simulink model "AED2D"  (R2018b)
settings: Solver=FixedStepAuto  StartTime=0.0  StopTime=Tfim  FixedStep=0.001  MaxStep=0.001  RelTol=1e-3
values from neighbouring files (symbols this model uses):
  D = DadosCGInercia(D)    [PlotGMax.m]    (also in S.mat = ; VooUnico.m; VooUnico6DOF.m)
  dados =     [S.mat]
  g = 9.8    [plot_exocet_6dof.m]
  M_CD = [8.341 8.24 8.141 8.043 7.946 7.851 7.76 7.674 7.595 7.523 7.46 7.4 ... (1365 elements, 21x5x13)]    [S.mat]
  M_CM = [42.757 43.119 43.498 43.905 44.357 44.839 45.319 45.775 46.191 46.536 46.769 46.963 ... (1365 elements, 21x5x13)]    [S.mat]
  M_CMQ = [-1543.746 -1552.906 -1559.915 -1565.64 -1570.662 -1573.443 -1572.931 -1569.859 -1564.198 -1553.449 -1535.22 -1514.504 ... (1365 elements, 21x5x13)]    [S.mat]
  M_CN = [-21.126 -21.088 -21.046 -20.997 -20.94 -20.877 -20.812 -20.749 -20.692 -20.644 -20.613 -20.587 ... (1365 elements, 21x5x13)]    [S.mat]
  R2D = 57.2957795131    [S.mat]    (also in VooUnico.m; VooUnico6DOF.m; plot6DOF.m; plot_exocet_6dof.m)
undefined symbols (not defined in the file or in its folder): AclnMax, AltCruz, anp, dist_manobra, Dlt_max, Dlt_max_roll, F_propB, F_propS, GanhoAtit, M_CMAD, M_CNAD, M_CNQ, manobra, Newton, ng, p0, phi0, psi0, psimaxAD, q0, r0, RampaMax, Raphson, sat_integAP, sigmaYmaxAD, sigmaZmaxAD, T_acel_k_ext, T_acel_k_int, T_at_k_ext, T_at_k_int, theta0, thetamaxAD, TLaser, Tresp, TTrav, vet_altitude, vet_Mach, vet_x_CG, Vxa0, Vya0, Vza0, Xa0, Ya0, Za0
libraries: simulink x11, sharedutil x4, aerolibasang x4, vrlib x3, shared6dof x2, aerolibatmos2 x1, dspmtrx3 x1
(part 1 of 2)
settings Model: Creator=carlberto-old  LastModifiedBy=carlberto-old
settings SFSimCC: SimUseLocalCustomCode=off
settings RTWCC: RTWUseLocalCustomCode=off

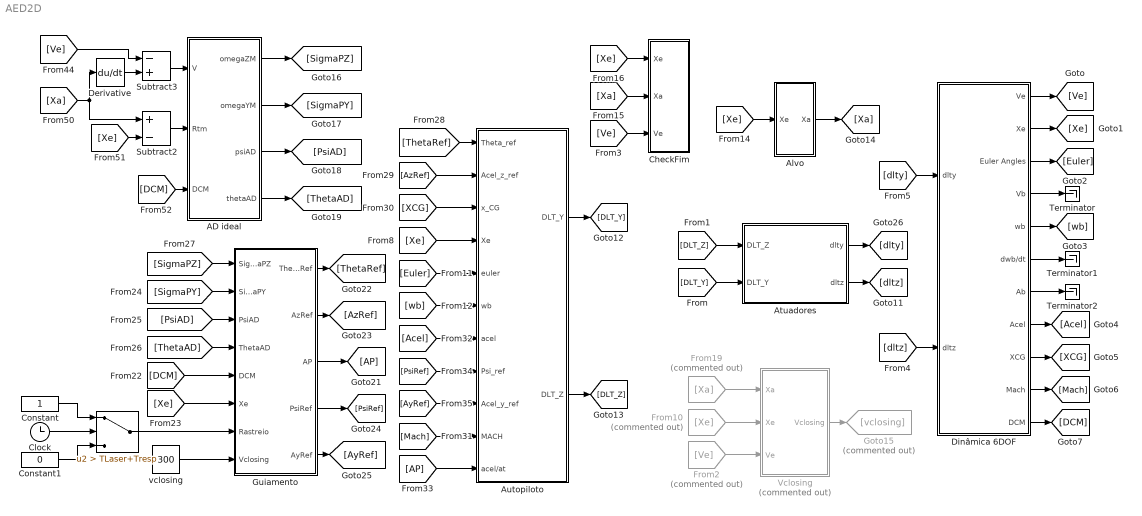
== system AED2D ==
  "  " : Switch  Criteria=u2 > Threshold  Threshold=TLaser+Tresp
  AD ideal : Subsystem
  Alvo : Subsystem
  Atuadores : Subsystem
  Autopiloto : Subsystem
  CheckFim : Subsystem
  Clock : Clock
  Constant : Constant
  Constant1 : Constant  Value=0
  Derivative : Derivative
  Dinâmica 6DOF : Subsystem
  From10 : From  Commented=on  GotoTag=Xe
  From19 : From  Commented=on  GotoTag=Xa
  From2 : From  Commented=on  GotoTag=Ve
  Goto15 : Goto  Commented=on  GotoTag=vclosing
  Guiamento : Subsystem
  Subtract2 : Sum  Inputs=+-
  Subtract3 : Sum  Inputs=-+
  Terminator : Terminator
  Terminator1 : Terminator
  Terminator2 : Terminator
  Vclosing : Subsystem  Commented=on
  vclosing : Constant  Value=300
  wires:
  [dltz] -> Dinâmica 6DOF/2(dltz)
  [DLT_Z] -> Atuadores/1(DLT_Z)
  [DLT_Y] -> Atuadores/2("DLT_Y ")
  Atuadores/2(dltz) -> [dltz]
  Atuadores/1("dlty ") -> [dlty]
  Dinâmica 6DOF/4(Vb) -> Terminator/1
  Dinâmica 6DOF/1(Ve) -> [Ve]
  Dinâmica 6DOF/2(Xe) -> [Xe]
  Dinâmica 6DOF/3(Euler Angles) -> [Euler]
  Dinâmica 6DOF/5(wb) -> [wb]
  Dinâmica 6DOF/8(Acel) -> [Acel]
  Dinâmica 6DOF/9(XCG) -> [XCG]
  Dinâmica 6DOF/10(Mach) -> [Mach]
  Dinâmica 6DOF/11(DCM) -> [DCM]
  Dinâmica 6DOF/6(dwb/dt) -> Terminator1/1
  Dinâmica 6DOF/7(Ab) -> Terminator2/1
  Clock/1 -> "  "/2
  [Xe] -> Subtract2/2
  AD ideal/3(psiAD) -> [PsiAD]
  Constant1/1 -> "  "/3
  [Acel] -> Autopiloto/7(acel)
  [Ve] -> Subtract3/1
  AD ideal/4(thetaAD) -> [ThetaAD]
  Subtract3/1 -> AD ideal/1(V)
  [Ve] -> CheckFim/3(Ve)
  AD ideal/1(omegaZM) -> [SigmaPZ]
  Subtract2/1 -> AD ideal/2(Rtm)
  [Xa] -> Subtract2/1, Derivative/1
  [AzRef] -> Autopiloto/2(Acel_z_ref)
  [AyRef] -> Autopiloto/9(Acel_y_ref)
  [Xe] -> Guiamento/6(Xe)
  Derivative/1 -> Subtract3/2
  Autopiloto/1(DLT_Y) -> [DLT_Y]
  vclosing/1 -> Guiamento/8(Vclosing)
  [AP] -> Autopiloto/11(acel/at)
  [Mach] -> Autopiloto/10(MACH)
  [PsiRef] -> Autopiloto/8(Psi_ref)
  Guiamento/4(PsiRef) -> [PsiRef]
  "  "/1 -> Guiamento/7(Rastreio)
  Guiamento/1(ThetaRef) -> [ThetaRef]
  Guiamento/2(AzRef) -> [AzRef]
  [DCM] -> Guiamento/5(DCM)
  Guiamento/5(AyRef) -> [AyRef]
  [Xa] -> CheckFim/2(Xa)
  [XCG] -> Autopiloto/3(x_CG)
  Autopiloto/2(DLT_Z) -> [DLT_Z]
  [Xe] -> Alvo/1(Xe)
  AD ideal/2(omegaYM) -> [SigmaPY]
  [ThetaAD] -> Guiamento/4(ThetaAD)
  [wb] -> Autopiloto/6(wb)
  [ThetaRef] -> Autopiloto/1(Theta_ref)
  [DCM] -> AD ideal/3(DCM)
  [Xe] -> Autopiloto/4(Xe)
  [Euler] -> Autopiloto/5(euler)
  Constant/1 -> "  "/1
  [SigmaPY] -> Guiamento/2(SigmaPY)
  Guiamento/3(AP) -> [AP]
  [Xe] -> CheckFim/1(Xe)
  [SigmaPZ] -> Guiamento/1(SigmaPZ)
  [PsiAD] -> Guiamento/3(PsiAD)
  From19/1 -> Vclosing/1(Xa)
  Alvo/1(Xa) -> [Xa]
  From10/1 -> Vclosing/2(Xe)
  From2/1 -> Vclosing/3(Ve)
  Vclosing/1(Vclosing) -> Goto15/1
  [dlty] -> Dinâmica 6DOF/1(dlty)

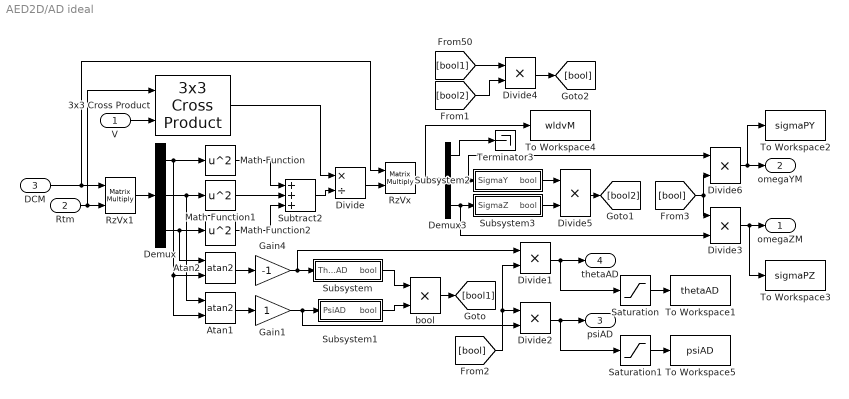
== system AED2D/AD ideal ==
  V : Inport
  Rtm : Inport  Port=2
  DCM : Inport  Port=3
  3x3 Cross Product : sharedutil/3x3 Cross Product
      settings: SourceProductBaseCode=AE
  Atan1 : Trigonometry  Operator=atan2
  Atan2 : Trigonometry  Operator=atan2
  Demux : Demux  Outputs=3
  Demux3 : Demux  Outputs=3
  Divide : Product  Inputs=*/
  Divide{1..6} (6 alike) : Product  Inputs=**
  Gain1 : Gain
  Gain4 : Gain  Gain=-1
  Math Function : Math  Operator=square  SaturateOnIntegerOverflow=on
  Math Function1 : Math  Operator=square  SaturateOnIntegerOverflow=on
  Math Function2 : Math  Operator=square  SaturateOnIntegerOverflow=on
  RzVx : Product  Multiplication=Matrix(*)  RndMeth=Zero
  RzVx1 : Product  Multiplication=Matrix(*)  RndMeth=Zero
  Saturation : Saturate  UpperLimit=thetamaxAD  LowerLimit=-thetamaxAD
  Saturation1 : Saturate  UpperLimit=psimaxAD  LowerLimit=-psimaxAD
  Subsystem : Subsystem
  Subsystem1 : Subsystem
  Subsystem2 : Subsystem
  Subsystem3 : Subsystem
  Subtract2 : Sum  Inputs=+++
  Terminator3 : Terminator
  To Workspace1 : ToWorkspace  VariableName=thetaAD  SaveFormat=Timeseries  SampleTime=-1
  To Workspace2 : ToWorkspace  VariableName=sigmaPY  SaveFormat=Timeseries  SampleTime=-1
  To Workspace3 : ToWorkspace  VariableName=sigmaPZ  SaveFormat=Timeseries  SampleTime=-1
  To Workspace4 : ToWorkspace  VariableName=wldvM  SaveFormat=Timeseries  SampleTime=-1
  To Workspace5 : ToWorkspace  VariableName=psiAD  SaveFormat=Timeseries  SampleTime=-1
  bool : Product
  omegaZM : Outport
  omegaYM : Outport  Port=2
  psiAD : Outport  Port=3
  thetaAD : Outport  Port=4
  wires:
  3x3 Cross Product/1 -> Divide/1
  Divide/1 -> RzVx/2
  Demux/2 -> Atan1/1, Math Function1/1
  Demux/3 -> Math Function2/1, Atan2/1
  Rtm/1 -> 3x3 Cross Product/1, RzVx1/2
  Math Function1/1 -> Subtract2/2
  Math Function/1 -> Subtract2/1
  Math Function2/1 -> Subtract2/3
  Subtract2/1 -> Divide/2
  DCM/1 -> RzVx1/1, RzVx/1
  RzVx/1 -> To Workspace4/1, Demux3/1
  V/1 -> 3x3 Cross Product/2
  Atan2/1 -> Gain4/1
  Atan1/1 -> Gain1/1
  Demux/1 -> Math Function/1, Atan1/2, Atan2/2
  Demux3/1 -> Terminator3/1
  Saturation/1 -> To Workspace1/1
  Saturation1/1 -> To Workspace5/1
  RzVx1/1 -> Demux/1
  Gain4/1 -> Subsystem/1(ThetaAD), Divide1/1
  Gain1/1 -> Divide2/2, Subsystem1/1(PsiAD)
  Divide1/1 -> thetaAD/1, Saturation/1
  Subsystem1/1(bool) -> bool/2
  Subsystem/1(bool) -> bool/1
  Divide2/1 -> psiAD/1, Saturation1/1
  Demux3/3 -> Divide3/2, Subsystem3/1(SigmaZ)
  Demux3/2 -> Subsystem2/1(SigmaY), Divide6/1
  Subsystem3/1(bool) -> Divide5/2
  Subsystem2/1(bool) -> Divide5/1
  bool/1 -> [bool1]
  Divide5/1 -> [bool2]
  [bool1] -> Divide4/1
  [bool2] -> Divide4/2
  Divide4/1 -> [bool]
  [bool] -> Divide1/2, Divide2/1
  Divide3/1 -> To Workspace3/1, omegaZM/1
  Divide6/1 -> To Workspace2/1, omegaYM/1
  [bool] -> Divide3/1, Divide6/2

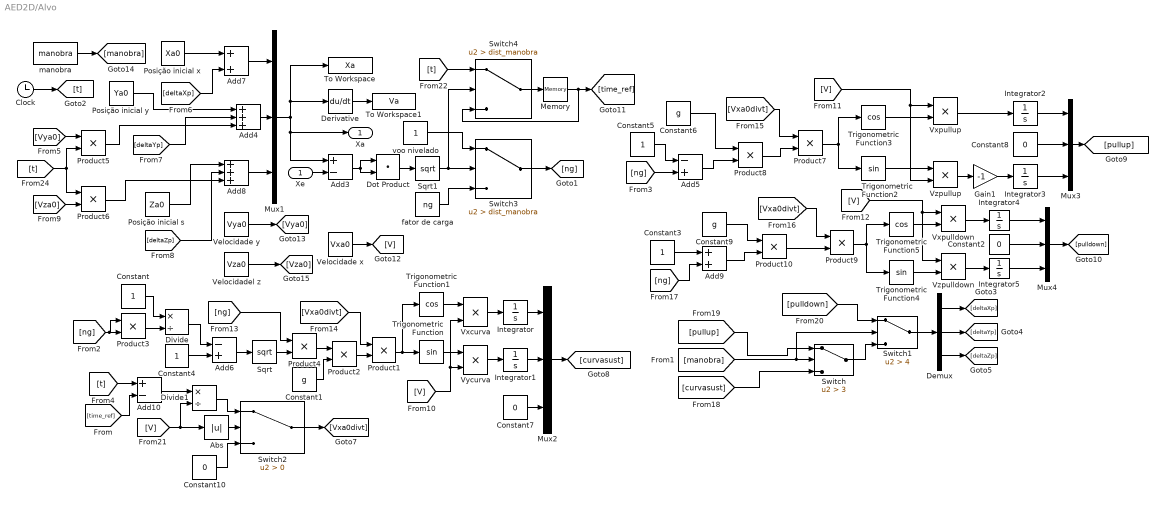
== system AED2D/Alvo ==
  Xe : Inport
  Abs : Abs
  Add10 : Sum  Inputs=+-
  Add3 : Sum  Inputs=+-
  Add4 : Sum  Inputs=+++
  Add5 : Sum  Inputs=-+
  Add6 : Sum  Inputs=-+
  Add7 : Sum
  Add8 : Sum  Inputs=+++
  Add9 : Sum
  Clock : Clock
  Constant{,3..5} (4 alike) : Constant
  Constant1 : Constant  Value=g
  Constant{2,7..8,10} (4 alike) : Constant  Value=0
  Constant6 : Constant  Value=g
  Constant9 : Constant  Value=g
  Demux : Demux  Outputs=3
  Derivative : Derivative
  Divide : Product  Inputs=*/
  Divide1 : Product  Inputs=*/
  Dot Product : DotProduct  InputSameDT=on  OutDataTypeStr=Inherit: Inherit via internal rule
  Gain1 : Gain  Gain=-1
  Integrator{,1..5} (6 alike) : Integrator
  Memory : Memory
  Mux{1..4} (4 alike) : Mux  Inputs=3
  Posição inicial s : Constant  Value=Za0
  Posição inicial x : Constant  Value=Xa0
  Posição inicial y : Constant  Value=Ya0
  Product{1..10} (10 alike) : Product
  Sqrt : Sqrt  SaturateOnIntegerOverflow=on
  Sqrt1 : Sqrt  SaturateOnIntegerOverflow=on
  Switch : Switch  Criteria=u2 > Threshold  Threshold=3
  Switch1 : Switch  Criteria=u2 > Threshold  Threshold=4
  Switch2 : Switch  Criteria=u2 > Threshold
  Switch3 : Switch  Criteria=u2 > Threshold  Threshold=dist_manobra
  Switch4 : Switch  Criteria=u2 > Threshold  Threshold=dist_manobra
  To Workspace : ToWorkspace  VariableName=Xa  SaveFormat=Timeseries  SampleTime=-1
  To Workspace1 : ToWorkspace  VariableName=Va  SaveFormat=Timeseries  SampleTime=-1
  Trigonometric Function : Trigonometry
  Trigonometric Function1 : Trigonometry  Operator=cos
  Trigonometric Function2 : Trigonometry
  Trigonometric Function3 : Trigonometry  Operator=cos
  Trigonometric Function4 : Trigonometry
  Trigonometric Function5 : Trigonometry  Operator=cos
  Velocidade x : Constant  Value=Vxa0
  "Velocidade y " : Constant  Value=Vya0
  Velocidadel z : Constant  Value=Vza0
  "Vxcurva " : Product
  Vxpulldown : Product
  Vxpullup : Product
  "Vycurva " : Product
  Vzpulldown : Product
  "Vzpullup " : Product
  fator de carga : Constant  Value=ng
  "manobra " : Constant  Value=manobra
  voo nivelado : Constant
  Xa : Outport
  wires:
  Demux/2 -> [deltaYp]
  Add4/1 -> Mux1/2
  Add9/1 -> Product10/2
  Product10/1 -> Product9/2
  Sqrt/1 -> Product4/2
  Integrator1/1 -> Mux2/2
  Add8/1 -> Mux1/3
  Posição inicial s/1 -> Add8/1
  Add7/1 -> Mux1/1
  Product4/1 -> Product2/1
  Trigonometric Function3/1 -> Vxpullup/2
  Product2/1 -> Product1/2
  Memory/1 -> [time_ref], Switch4/3
  [Vya0] -> Product5/1
  [deltaYp] -> Add4/2
  Constant4/1 -> Add6/2
  Constant9/1 -> Product10/1
  Product5/1 -> Add4/3
  "Vxcurva "/1 -> Integrator/1
  Product6/1 -> Add8/3
  Integrator2/1 -> Mux3/1
  "manobra "/1 -> [manobra]
  [Vza0] -> Product6/2
  Posição inicial x/1 -> Add7/1
  [ng] -> Product4/1
  Velocidade x/1 -> [V]
  Integrator4/1 -> Mux4/1
  [V] -> Divide1/2, Abs/1
  "Vzpullup "/1 -> Gain1/1
  Product1/1 -> Trigonometric Function/1, Trigonometric Function1/1
  Gain1/1 -> Integrator3/1
  [V] -> "Vzpullup "/2, Vxpullup/1
  "Vycurva "/1 -> Integrator1/1
  Add6/1 -> Sqrt/1
  [V] -> "Vxcurva "/2, "Vycurva "/2
  fator de carga/1 -> Switch3/3
  Trigonometric Function4/1 -> Vzpulldown/2
  Mux4/1 -> [pulldown]
  Add10/1 -> Divide1/1
  Mux1/1 -> To Workspace/1, Derivative/1, Xa/1, Add3/1
  [Vxa0divt] -> Product1/1
  Demux/3 -> [deltaZp]
  [ng] -> Add9/2
  [time_ref] -> Add10/2
  [V] -> Vzpulldown/1, Vxpulldown/1
  Constant5/1 -> Add5/1
  [ng] -> Add5/2
  Clock/1 -> [t]
  Add3/1 -> Dot Product/2, Dot Product/1
  [ng] -> Product3/1, Product3/2
  [deltaXp] -> Add7/2
  [Vxa0divt] -> Product9/1
  Product9/1 -> Trigonometric Function5/1, Trigonometric Function4/1
  Posição inicial y/1 -> Add4/1
  Trigonometric Function5/1 -> Vxpulldown/2
  Vxpulldown/1 -> Integrator4/1
  voo nivelado/1 -> Switch3/1
  Xe/1 -> Add3/2
  Constant10/1 -> Switch2/3
  Constant7/1 -> Mux2/3
  Mux2/1 -> [curvasust]
  Demux/1 -> [deltaXp]
  Sqrt1/1 -> Switch3/2, Switch4/2
  Constant1/1 -> Product2/2
  Switch/1 -> Switch1/3
  [deltaZp] -> Add8/2
  Product8/1 -> Product7/2
  [curvasust] -> Switch/3
  Vzpulldown/1 -> Integrator5/1
  Add5/1 -> Product8/2
  Velocidadel z/1 -> [Vza0]
  Switch3/1 -> [ng]
  Constant/1 -> Divide/1
  Vxpullup/1 -> Integrator2/1
  Constant6/1 -> Product8/1
  [t] -> Switch4/1
  Constant2/1 -> Mux4/2
  Integrator/1 -> Mux2/1
  [t] -> Product6/1, Product5/2
  [Vxa0divt] -> Product7/1
  Trigonometric Function1/1 -> "Vxcurva "/1
  [manobra] -> Switch1/2, Switch/2
  Integrator5/1 -> Mux4/3
  Constant3/1 -> Add9/1
  Divide1/1 -> Switch2/1
  Mux3/1 -> [pullup]
  Trigonometric Function/1 -> "Vycurva "/1
  Product3/1 -> Divide/2
  Trigonometric Function2/1 -> "Vzpullup "/1
  Abs/1 -> Switch2/2
  Product7/1 -> Trigonometric Function3/1, Trigonometric Function2/1
  Divide/1 -> Add6/1
  [pulldown] -> Switch1/1
  [t] -> Add10/1
  [pullup] -> Switch/1
  Dot Product/1 -> Sqrt1/1
  Switch4/1 -> Memory/1
  Switch2/1 -> [Vxa0divt]
  Derivative/1 -> To Workspace1/1
  "Velocidade y "/1 -> [Vya0]
  Constant8/1 -> Mux3/2
  Switch1/1 -> Demux/1
  Integrator3/1 -> Mux3/3

== system AED2D/Atuadores ==
  DLT_Z : Inport
  "DLT_Y " : Inport  Port=2
  Add : Sum  Commented=on
  Gain : Gain  Commented=on  Gain=1/sqrt(2)
  Saturation1 : Saturate  UpperLimit=Dlt_max  LowerLimit=-Dlt_max
  Saturation2 : Saturate  UpperLimit=Dlt_max  LowerLimit=-Dlt_max
  Transfer Fcn1 : TransferFcn  Numerator=[300]  Denominator=[1 300]
  Transfer Fcn2 : TransferFcn  Numerator=[300]  Denominator=[1 300]
  "dlty " : Outport
  dltz : Outport  Port=2
  wires:
  Transfer Fcn1/1 -> Saturation1/1
  Saturation1/1 -> "dlty "/1
  Transfer Fcn2/1 -> Saturation2/1
  Saturation2/1 -> dltz/1
  Add/1 -> Gain/1
  "DLT_Y "/1 -> Transfer Fcn1/1
  DLT_Z/1 -> Transfer Fcn2/1

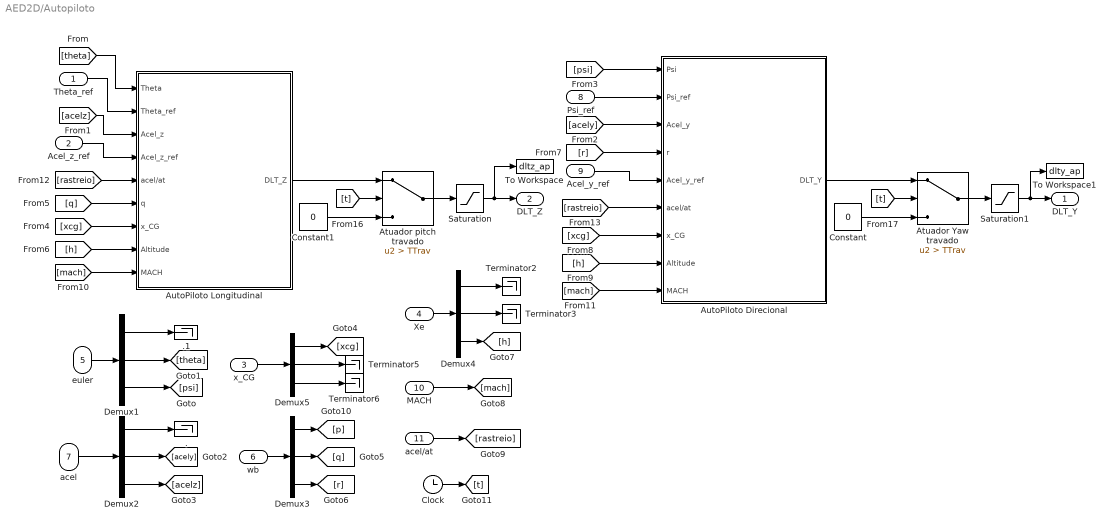
== system AED2D/Autopiloto ==
  Theta_ref : Inport
  Acel_z_ref : Inport  Port=2
  x_CG : Inport  Port=3
  Xe : Inport  Port=4
  euler : Inport  Port=5
  wb : Inport  Port=6
  acel : Inport  Port=7
  Psi_ref : Inport  Port=8
  Acel_y_ref : Inport  Port=9
  MACH : Inport  Port=10
  acel/at : Inport  Port=11
  . : Terminator
  .1 : Terminator
  Atuador Yaw travado : Switch  Criteria=u2 > Threshold  Threshold=TTrav
  Atuador pitch travado : Switch  Criteria=u2 > Threshold  Threshold=TTrav
  AutoPiloto Direcional : Subsystem
  AutoPiloto Longitudinal : Subsystem
  Clock : Clock
  Constant : Constant  Value=0
  Constant1 : Constant  Value=0
  Demux{1..5} (5 alike) : Demux  Outputs=3
  Saturation : Saturate  UpperLimit=Dlt_max  LowerLimit=-Dlt_max
  Saturation1 : Saturate  UpperLimit=Dlt_max  LowerLimit=-Dlt_max
  Terminator{2..3,5..6} (4 alike) : Terminator
  To Workspace : ToWorkspace  VariableName=dltz_ap  SaveFormat=Timeseries  SampleTime=-1
  To Workspace1 : ToWorkspace  VariableName=dlty_ap  SaveFormat=Timeseries  SampleTime=-1
  DLT_Y : Outport
  DLT_Z : Outport  Port=2
  wires:
  Theta_ref/1 -> AutoPiloto Longitudinal/2(Theta_ref)
  acel/1 -> Demux2/1
  wb/1 -> Demux3/1
  Xe/1 -> Demux4/1
  euler/1 -> Demux1/1
  Demux2/1 -> ./1
  Demux4/1 -> Terminator2/1
  Demux4/2 -> Terminator3/1
  Demux3/1 -> [p]
  Psi_ref/1 -> AutoPiloto Direcional/2(Psi_ref)
  Acel_y_ref/1 -> AutoPiloto Direcional/5(Acel_y_ref)
  Acel_z_ref/1 -> AutoPiloto Longitudinal/4(Acel_z_ref)
  Demux1/1 -> .1/1
  x_CG/1 -> Demux5/1
  Demux5/2 -> Terminator5/1
  Demux5/3 -> Terminator6/1
  AutoPiloto Longitudinal/1(DLT_Z) -> Atuador pitch travado/1
  Constant/1 -> Atuador Yaw travado/3
  AutoPiloto Direcional/1(DLT_Y) -> Atuador Yaw travado/1
  Demux1/2 -> [theta]
  Demux1/3 -> [psi]
  [theta] -> AutoPiloto Longitudinal/1(Theta)
  Demux2/3 -> [acelz]
  Demux2/2 -> [acely]
  [acelz] -> AutoPiloto Longitudinal/3(Acel_z)
  [acely] -> AutoPiloto Direcional/3(Acel_y)
  [psi] -> AutoPiloto Direcional/1(Psi)
  Demux5/1 -> [xcg]
  [xcg] -> AutoPiloto Longitudinal/7(x_CG)
  Demux3/2 -> [q]
  Demux3/3 -> [r]
  [q] -> AutoPiloto Longitudinal/6(q)
  Demux4/3 -> [h]
  [h] -> AutoPiloto Longitudinal/8(Altitude)
  [r] -> AutoPiloto Direcional/4(r)
  [xcg] -> AutoPiloto Direcional/7(x_CG)
  [h] -> AutoPiloto Direcional/8(Altitude)
  MACH/1 -> [mach]
  [mach] -> AutoPiloto Longitudinal/9(MACH)
  [mach] -> AutoPiloto Direcional/9(MACH)
  acel/at/1 -> [rastreio]
  [rastreio] -> AutoPiloto Longitudinal/5(acel/at)
  [rastreio] -> AutoPiloto Direcional/6(acel/at)
  Constant1/1 -> Atuador pitch travado/3
  Atuador pitch travado/1 -> Saturation/1
  Saturation/1 -> To Workspace/1, DLT_Z/1
  Atuador Yaw travado/1 -> Saturation1/1
  Saturation1/1 -> DLT_Y/1, To Workspace1/1
  Clock/1 -> [t]
  [t] -> Atuador pitch travado/2
  [t] -> Atuador Yaw travado/2

== system AED2D/CheckFim ==
  Xe : Inport
  Xa : Inport  Port=2
  Ve : Inport  Port=3
  Add : Sum  Inputs=+-
  Compare To Constant1 : simulink/Logic and Bit Operations/Compare To Constant  relop=>  const=0  OutDataTypeStr=boolean
  Compare To Zero : simulink/Logic and Bit Operations/Compare To Zero  relop=>=  OutDataTypeStr=boolean
  Demux : Demux  Outputs=3
  Dot Product : DotProduct  InputSameDT=on  OutDataTypeStr=Inherit: Inherit via internal rule
  Normalize Vector : vrlib/Utilities/Normalize Vector  maxzero=0
      settings: SourceProductName=Simulink 3D Animation  SourceProductBaseCode=VR
  Normalize Vector1 : vrlib/Utilities/Normalize Vector  maxzero=0
      settings: SourceProductName=Simulink 3D Animation  SourceProductBaseCode=VR
  Stop Simulation : Stop
  Stop Simulation2 : Stop
  Terminator2 : Terminator
  Terminator3 : Terminator
  wires:
  Xe/1 -> Add/1, Demux/1
  Demux/1 -> Terminator2/1
  Demux/2 -> Terminator3/1
  Compare To Zero/1 -> Stop Simulation/1
  Demux/3 -> Compare To Zero/1
  Xa/1 -> Add/2
  Add/1 -> Normalize Vector/1
  Normalize Vector/1 -> Dot Product/1
  Normalize Vector1/1 -> Dot Product/2
  Dot Product/1 -> Compare To Constant1/1
  Ve/1 -> Normalize Vector1/1
  Compare To Constant1/1 -> Stop Simulation2/1

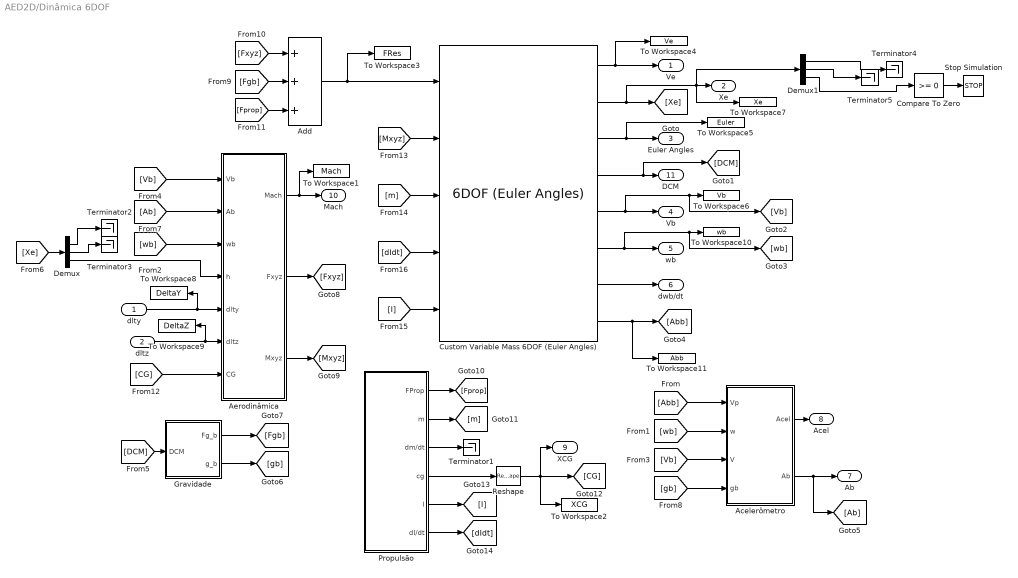
== system AED2D/Dinâmica 6DOF ==
  dlty : Inport
  dltz : Inport  Port=2
  Acelerômetro : Subsystem
  Add : Sum  Inputs=+++
  Aerodinâmica : Subsystem
  Compare To Zero : simulink/Logic and Bit Operations/Compare To Zero  relop=>=  OutDataTypeStr=boolean
  Custom Variable Mass 6DOF (Euler Angles) : shared6dof/6DOF (Euler Angles)  units=Metric (MKS)  mtype=Custom Variable  rep=Euler Angles  xme_0=[0 0 -D.Alt0]  Vm_0=[D.U 0 0]  eul_0="[phi0  theta0   psi0]"  pm_0=[p0 q0 r0]  mass_0=1.0  mass_e=0.5  mass_f=2.0  inertia=eye(3)  inertia_e=eye(3)  inertia_f=2*eye(3)  k_quat=1.0  vre_flag=off  abi_flag=off  aMode=aMode  xme_statename=''  Vm_statename=''  eul_statename=''  quat_statename=''  pm_statename=''  mass_statename=''
      settings: SourceProductBaseCode=AE
  Demux : Demux  Outputs=3
  Demux1 : Demux  Outputs=3
  Gravidade : Subsystem
  Propulsão : Subsystem
  Reshape : Reshape
  Stop Simulation : Stop
  Terminator{1..5} (5 alike) : Terminator
  To Workspace1 : ToWorkspace  VariableName=Mach  SaveFormat=Timeseries  SampleTime=-1
  To Workspace10 : ToWorkspace  VariableName=wb  SaveFormat=Timeseries  SampleTime=-1
  To Workspace11 : ToWorkspace  VariableName=Abb  SaveFormat=Timeseries  SampleTime=-1
  To Workspace2 : ToWorkspace  VariableName=XCG  SaveFormat=Timeseries  SampleTime=-1
  To Workspace3 : ToWorkspace  VariableName=FRes  SaveFormat=Timeseries  SampleTime=-1
  To Workspace4 : ToWorkspace  VariableName=Ve  SaveFormat=Timeseries  SampleTime=-1
  To Workspace5 : ToWorkspace  VariableName=Euler  SaveFormat=Timeseries  SampleTime=-1
  To Workspace6 : ToWorkspace  VariableName=Vb  SaveFormat=Timeseries  SampleTime=-1
  To Workspace7 : ToWorkspace  VariableName=Xe  SaveFormat=Timeseries  SampleTime=-1
  To Workspace8 : ToWorkspace  VariableName=DeltaY  SaveFormat=Timeseries  SampleTime=-1
  To Workspace9 : ToWorkspace  VariableName=DeltaZ  SaveFormat=Timeseries  SampleTime=-1
  Ve : Outport
  Xe : Outport  Port=2
  Euler Angles : Outport  Port=3
  Vb : Outport  Port=4
  wb : Outport  Port=5
  dwb/dt : Outport  Port=6
  Ab : Outport  Port=7
  Acel : Outport  Port=8
  XCG : Outport  Port=9
  Mach : Outport  Port=10
  DCM : Outport  Port=11
  wires:
  dltz/1 -> Aerodinâmica/6(dltz), To Workspace9/1
  Custom Variable Mass 6DOF (Euler Angles)/1 -> Ve/1, To Workspace4/1
  Custom Variable Mass 6DOF (Euler Angles)/3 -> Euler Angles/1, To Workspace5/1
  Custom Variable Mass 6DOF (Euler Angles)/7 -> dwb/dt/1
  Demux/1 -> Terminator2/1
  dlty/1 -> To Workspace8/1, Aerodinâmica/5(dlty)
  Demux/2 -> Terminator3/1
  Custom Variable Mass 6DOF (Euler Angles)/5 -> Vb/1, [Vb], To Workspace6/1
  Add/1 -> Custom Variable Mass 6DOF (Euler Angles)/1, To Workspace3/1
  Custom Variable Mass 6DOF (Euler Angles)/4 -> [DCM], DCM/1
  Demux/3 -> Aerodinâmica/4(h)
  Aerodinâmica/1(Mach) -> To Workspace1/1, Mach/1
  Propulsão/3(dm/dt) -> Terminator1/1
  Reshape/1 -> XCG/1, To Workspace2/1, [CG]
  Acelerômetro/1(Acel) -> Acel/1
  Propulsão/4(cg) -> Reshape/1
  [Abb] -> Acelerômetro/1(Vp)
  [wb] -> Acelerômetro/2(w)
  [wb] -> Aerodinâmica/3(wb)
  [Vb] -> Acelerômetro/3(V)
  [Vb] -> Aerodinâmica/1(Vb)
  [DCM] -> Gravidade/1(DCM)
  [Xe] -> Demux/1
  Acelerômetro/2(Ab) -> [Ab], Ab/1
  [Ab] -> Aerodinâmica/2(Ab)
  [gb] -> Acelerômetro/4(gb)
  Gravidade/2(g_b) -> [gb]
  Gravidade/1(Fg_b) -> [Fgb]
  [Fgb] -> Add/2
  [Fxyz] -> Add/1
  Aerodinâmica/2(Fxyz) -> [Fxyz]
  Aerodinâmica/3(Mxyz) -> [Mxyz]
  [CG] -> Aerodinâmica/7(CG)
  Propulsão/1(FProp) -> [Fprop]
  Propulsão/2(m) -> [m]
  Propulsão/5(I) -> [I]
  Propulsão/6(dI/dt) -> [dIdt]
  [Mxyz] -> Custom Variable Mass 6DOF (Euler Angles)/2
  [m] -> Custom Variable Mass 6DOF (Euler Angles)/3
  [I] -> Custom Variable Mass 6DOF (Euler Angles)/5
  [dIdt] -> Custom Variable Mass 6DOF (Euler Angles)/4
  Custom Variable Mass 6DOF (Euler Angles)/6 -> [wb], To Workspace10/1, wb/1
  Custom Variable Mass 6DOF (Euler Angles)/8 -> To Workspace11/1, [Abb]
  Demux1/1 -> Terminator4/1
  Custom Variable Mass 6DOF (Euler Angles)/2 -> Demux1/1, To Workspace7/1, Xe/1, [Xe]
  Compare To Zero/1 -> Stop Simulation/1
  Demux1/2 -> Terminator5/1
  Demux1/3 -> Compare To Zero/1
  [Fprop] -> Add/3

== system AED2D/Guiamento ==
  SigmaPZ : Inport
  SigmaPY : Inport  Port=2
  PsiAD : Inport  Port=3
  ThetaAD : Inport  Port=4
  DCM : Inport  Port=5
  Xe : Inport  Port=6
  Rastreio : Inport  Port=7
  Vclosing : Inport  Port=8
  Controle de Atitude : Subsystem
  "Navegação Proporcional " : Subsystem
  Saturation : Saturate  UpperLimit=AclnMax  LowerLimit=-AclnMax
  Saturation1 : Saturate  UpperLimit=AclnMax  LowerLimit=-AclnMax
  To Workspace1 : ToWorkspace  VariableName=Guiamento  SaveFormat=Timeseries  SampleTime=-1
  To Workspace2 : ToWorkspace  VariableName=AzRef  SaveFormat=Timeseries  SampleTime=-1
  To Workspace3 : ToWorkspace  VariableName=AyRef  SaveFormat=Timeseries  SampleTime=-1
  ThetaRef : Outport
  AzRef : Outport  Port=2
  AP : Outport  Port=3
  PsiRef : Outport  Port=4
  AyRef : Outport  Port=5
  wires:
  Controle de Atitude/2(ThetaRef) -> ThetaRef/1
  SigmaPZ/1 -> "Navegação Proporcional "/1(SigmaPZ)
  SigmaPY/1 -> "Navegação Proporcional "/2(SigmaPY)
  PsiAD/1 -> "Navegação Proporcional "/3(PsiAD)
  ThetaAD/1 -> "Navegação Proporcional "/4(ThetaAD)
  DCM/1 -> "Navegação Proporcional "/5(CMI)
  Rastreio/1 -> To Workspace1/1, AP/1, [rastreio]
  Controle de Atitude/1(psiREF) -> PsiRef/1
  Xe/1 -> Controle de Atitude/1(Xe)
  Vclosing/1 -> "Navegação Proporcional "/7(Vclosing)
  [rastreio] -> "Navegação Proporcional "/6(AP)
  [rastreio] -> Controle de Atitude/2(AP)
  Saturation/1 -> To Workspace2/1
  Saturation1/1 -> To Workspace3/1
  "Navegação Proporcional "/1(AzRef) -> AzRef/1, Saturation/1
  "Navegação Proporcional "/2(AyRef) -> AyRef/1, Saturation1/1

== system AED2D/Vclosing ==
  Xa : Inport
  Xe : Inport  Port=2
  Ve : Inport  Port=3
  Derivative : Derivative
  Dot Product : DotProduct  InputSameDT=on  OutDataTypeStr=Inherit: Inherit via internal rule
  Dot Product1 : DotProduct  InputSameDT=on  OutDataTypeStr=Inherit: Inherit via internal rule
  Normalize Vector : vrlib/Utilities/Normalize Vector  maxzero=0
      settings: SourceProductName=Simulink 3D Animation  SourceProductBaseCode=VR
  Subtract : Sum  Inputs=-+
  Subtract1 : Sum  Inputs=+-
  To Workspace : ToWorkspace  VariableName=Vclosing  SaveFormat=Timeseries  SampleTime=-1
  Vclosing : Outport
  wires:
  Xa/1 -> Subtract/2, Derivative/1
  Subtract/1 -> Normalize Vector/1
  Subtract1/1 -> Vclosing/1, To Workspace/1
  Ve/1 -> Dot Product1/1
  Dot Product1/1 -> Subtract1/1
  Dot Product/1 -> Subtract1/2
  Xe/1 -> Subtract/1
  Derivative/1 -> Dot Product/2
  Normalize Vector/1 -> Dot Product1/2, Dot Product/1

== system AED2D/AD ideal/Subsystem ==
  ThetaAD : Inport
  Abs : Abs
  Clock : Clock
  Compare To Constant : simulink/Logic and Bit Operations/Compare To Constant  relop=<  const=thetamaxAD  OutDataTypeStr=uint8
  Constant : Constant  Value=0
  Constant1 : Constant
  Memory : Memory  InitialCondition=1
  Switch : Switch  Criteria=u2 > Threshold
  Switch1 : Switch  Criteria=u2 > Threshold  Threshold=TLaser+Tresp
  bool : Outport
  wires:
  Memory/1 -> Switch/2
  Compare To Constant/1 -> Switch1/1
  Clock/1 -> Switch1/2
  Switch1/1 -> Switch/1
  Constant/1 -> Switch/3
  Abs/1 -> Compare To Constant/1
  Constant1/1 -> Switch1/3
  Switch/1 -> Memory/1, bool/1
  ThetaAD/1 -> Abs/1

== system AED2D/AD ideal/Subsystem1 ==
  PsiAD : Inport
  Abs : Abs
  Clock : Clock
  Compare To Constant : simulink/Logic and Bit Operations/Compare To Constant  relop=<  const=psimaxAD  OutDataTypeStr=uint8
  Constant : Constant  Value=0
  Constant1 : Constant
  Memory : Memory  InitialCondition=1
  Switch : Switch  Criteria=u2 > Threshold
  Switch1 : Switch  Criteria=u2 > Threshold  Threshold=TLaser+Tresp
  bool : Outport
  wires:
  Memory/1 -> Switch/2
  Compare To Constant/1 -> Switch1/1
  Clock/1 -> Switch1/2
  Switch1/1 -> Switch/1
  Constant/1 -> Switch/3
  Abs/1 -> Compare To Constant/1
  Constant1/1 -> Switch1/3
  Switch/1 -> Memory/1, bool/1
  PsiAD/1 -> Abs/1

== system AED2D/AD ideal/Subsystem2 ==
  SigmaY : Inport
  Abs : Abs
  Clock : Clock
  Compare To Constant : simulink/Logic and Bit Operations/Compare To Constant  relop=<  const=sigmaYmaxAD  OutDataTypeStr=uint8
  Constant : Constant  Value=0
  Constant1 : Constant
  Memory : Memory  InitialCondition=1
  Switch : Switch  Criteria=u2 > Threshold
  Switch1 : Switch  Criteria=u2 > Threshold  Threshold=TLaser+Tresp
  bool : Outport
  wires:
  Memory/1 -> Switch/2
  Compare To Constant/1 -> Switch1/1
  Clock/1 -> Switch1/2
  Switch1/1 -> Switch/1
  Constant/1 -> Switch/3
  Abs/1 -> Compare To Constant/1
  Constant1/1 -> Switch1/3
  Switch/1 -> Memory/1, bool/1
  SigmaY/1 -> Abs/1

== system AED2D/AD ideal/Subsystem3 ==
  SigmaZ : Inport
  Abs : Abs
  Clock : Clock
  Compare To Constant : simulink/Logic and Bit Operations/Compare To Constant  relop=<  const=sigmaZmaxAD  OutDataTypeStr=uint8
  Constant : Constant  Value=0
  Constant1 : Constant
  Memory : Memory  InitialCondition=1
  Switch : Switch  Criteria=u2 > Threshold
  Switch1 : Switch  Criteria=u2 > Threshold  Threshold=TLaser+Tresp
  bool : Outport
  wires:
  Memory/1 -> Switch/2
  Compare To Constant/1 -> Switch1/1
  Clock/1 -> Switch1/2
  Switch1/1 -> Switch/1
  Constant/1 -> Switch/3
  Abs/1 -> Compare To Constant/1
  Constant1/1 -> Switch1/3
  Switch/1 -> Memory/1, bool/1
  SigmaZ/1 -> Abs/1

== system AED2D/Autopiloto/AutoPiloto Direcional ==
  Psi : Inport
  Psi_ref : Inport  Port=2
  Acel_y : Inport  Port=3
  r : Inport  Port=4
  Acel_y_ref : Inport  Port=5
  acel/at : Inport  Port=6
  x_CG : Inport  Port=7
  Altitude : Inport  Port=8
  MACH : Inport  Port=9
  Rastreador de aceleração : Subsystem
  Rastreador de atitude : Subsystem
  Switch : Switch  Criteria=u2 > Threshold
  DLT_Y : Outport
  wires:
  Switch/1 -> DLT_Y/1
  Psi/1 -> Rastreador de atitude/5(Psi)
  Rastreador de atitude/1(DLTYC_atitude) -> Switch/3
  Acel_y/1 -> Rastreador de aceleração/1(Acel_y)
  Acel_y_ref/1 -> Rastreador de aceleração/2(Acel_y_ref)
  Rastreador de aceleração/1(DLTYC_acel) -> Switch/1
  acel/at/1 -> [acel]
  r/1 -> [r]
  x_CG/1 -> [xcg]
  Altitude/1 -> [altitude]
  MACH/1 -> [mach]
  [r] -> Rastreador de aceleração/3(r)
  [xcg] -> Rastreador de aceleração/4(x_CG)
  [altitude] -> Rastreador de aceleração/5(Altitude)
  [mach] -> Rastreador de aceleração/6(MACH)
  [r] -> Rastreador de atitude/1(r)
  [xcg] -> Rastreador de atitude/2(x_CG)
  [altitude] -> Rastreador de atitude/3(Altitude)
  [mach] -> Rastreador de atitude/4(MACH)
  [acel] -> Rastreador de aceleração/7(acel/at)
  [acel] -> Switch/2
  Psi_ref/1 -> Rastreador de atitude/6(Psi_ref)

== system AED2D/Autopiloto/AutoPiloto Longitudinal ==
  Theta : Inport
  Theta_ref : Inport  Port=2
  Acel_z : Inport  Port=3
  Acel_z_ref : Inport  Port=4
  acel/at : Inport  Port=5
  q : Inport  Port=6
  x_CG : Inport  Port=7
  Altitude : Inport  Port=8
  MACH : Inport  Port=9
  Rastreador de aceleração : Subsystem
  Rastreador de atitude : Subsystem
  Seleção entre Rastreadores : Switch  Criteria=u2 > Threshold
  DLT_Z : Outport
  wires:
  Theta/1 -> Rastreador de atitude/1(Theta)
  Theta_ref/1 -> Rastreador de atitude/2(Theta_ref)
  Acel_z/1 -> Rastreador de aceleração/1(Acel_z)
  Acel_z_ref/1 -> Rastreador de aceleração/2(Acel_z_ref)
  acel/at/1 -> [acel]
  Seleção entre Rastreadores/1 -> DLT_Z/1
  [q] -> Rastreador de aceleração/3(q)
  [xcg] -> Rastreador de aceleração/4(x_CG)
  [altitude] -> Rastreador de aceleração/5(Altitude)
  [mach] -> Rastreador de aceleração/6(MACH)
  [q] -> Rastreador de atitude/3(q)
  [xcg] -> Rastreador de atitude/4(x_CG)
  [altitude] -> Rastreador de atitude/5(Altitude)
  [mach] -> Rastreador de atitude/6(MACH)
  x_CG/1 -> [xcg]
  q/1 -> [q]
  MACH/1 -> [mach]
  Altitude/1 -> [altitude]
  Rastreador de aceleração/1(DLTZC_acel) -> Seleção entre Rastreadores/1
  Rastreador de atitude/1(DLTZC_atitude) -> Seleção entre Rastreadores/3
  [acel] -> Rastreador de aceleração/7(acel/at)
  [acel] -> Seleção entre Rastreadores/2

== system AED2D/Dinâmica 6DOF/Acelerômetro ==
  Vp : Inport
  w : Inport  Port=2
  V : Inport  Port=3
  gb : Inport  Port=4
  Add1 : Sum
  Add2 : Sum  Inputs=+-
  To Workspace4 : ToWorkspace  VariableName=Acel  SaveFormat=Timeseries  SampleTime=-1
  To Workspace5 : ToWorkspace  VariableName=Ab  SaveFormat=Timeseries  SampleTime=-1
  w x V : sharedutil/3x3 Cross Product
      settings: SourceProductBaseCode=AE
  Acel : Outport
  Ab : Outport  Port=2
  wires:
  V/1 -> w x V/2
  w/1 -> w x V/1
  w x V/1 -> Add1/2
  Vp/1 -> Add1/1
  Add1/1 -> Add2/1, Ab/1, To Workspace5/1
  gb/1 -> Add2/2
  Add2/1 -> To Workspace4/1, Acel/1

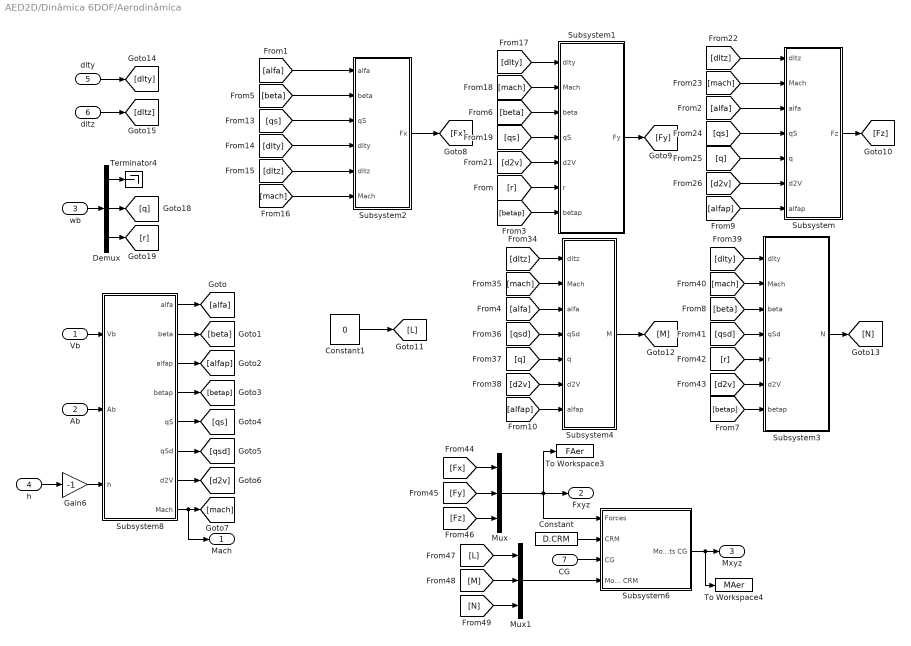
== system AED2D/Dinâmica 6DOF/Aerodinâmica ==
  Vb : Inport
  Ab : Inport  Port=2
  wb : Inport  Port=3
  h : Inport  Port=4
  dlty : Inport  Port=5
  dltz : Inport  Port=6
  CG : Inport  Port=7
  Constant : Constant  Value=D.CRM
  Constant1 : Constant  Value=0
  Demux : Demux  Outputs=3
  Gain6 : Gain  Gain=-1
  Mux : Mux  Inputs=3
  Mux1 : Mux  Inputs=3
  Subsystem : Subsystem
  Subsystem1 : Subsystem
  Subsystem2 : Subsystem
  Subsystem3 : Subsystem
  Subsystem4 : Subsystem
  Subsystem6 : Subsystem
  Subsystem8 : Subsystem
  Terminator4 : Terminator
  To Workspace3 : ToWorkspace  VariableName=FAer  SaveFormat=Timeseries  SampleTime=-1
  To Workspace4 : ToWorkspace  VariableName=MAer  SaveFormat=Timeseries  SampleTime=-1
  Mach : Outport
  Fxyz : Outport  Port=2
  Mxyz : Outport  Port=3
  wires:
  h/1 -> Gain6/1
  Mux1/1 -> Subsystem6/4(Moments CRM)
  Mux/1 -> Subsystem6/1(Forces), To Workspace3/1, Fxyz/1
  wb/1 -> Demux/1
  Vb/1 -> Subsystem8/1(Vb)
  Ab/1 -> Subsystem8/2(Ab)
  Gain6/1 -> Subsystem8/3(h)
  CG/1 -> Subsystem6/3(CG)
  Constant/1 -> Subsystem6/2(CRM)
  Subsystem6/1(Moments CG) -> Mxyz/1, To Workspace4/1
  Subsystem8/1(alfa) -> [alfa]
  [alfa] -> Subsystem2/1(alfa)
  [alfa] -> Subsystem/3(alfa)
  [alfa] -> Subsystem4/3(alfa)
  Subsystem8/2(beta) -> [beta]
  [beta] -> Subsystem2/2(beta)
  [beta] -> Subsystem1/3(beta)
  [beta] -> Subsystem3/3(beta)
  Subsystem8/3(alfap) -> [alfap]
  [alfap] -> Subsystem/7(alfap)
  [alfap] -> Subsystem4/7(alfap)
  Subsystem8/4(betap) -> [betap]
  Subsystem8/5(qS) -> [qs]
  Subsystem8/6(qSd) -> [qsd]
  Subsystem8/7(d2V) -> [d2v]
  Subsystem8/8(Mach) -> Mach/1, [mach]
  [qs] -> Subsystem2/3(qS)
  [dlty] -> Subsystem2/4(dlty)
  [dltz] -> Subsystem2/5(dltz)
  [mach] -> Subsystem2/6("Mach ")
  Subsystem2/1(Fx) -> [Fx]
  [dlty] -> Subsystem1/1("dlty ")
  [mach] -> Subsystem1/2(Mach)
  [qs] -> Subsystem1/4(qS)
  [d2v] -> Subsystem1/5(d2V)
  Subsystem1/1(Fy) -> [Fy]
  [dltz] -> Subsystem/1(dltz)
  [mach] -> Subsystem/2("Mach ")
  [qs] -> Subsystem/4(qS)
  [q] -> Subsystem/5(q)
  [d2v] -> Subsystem/6(d2V)
  Subsystem/1(Fz) -> [Fz]
  [dltz] -> Subsystem4/1(dltz)
  [mach] -> Subsystem4/2(Mach)
  [qsd] -> Subsystem4/4(qSd)
  [q] -> Subsystem4/5(q)
  [d2v] -> Subsystem4/6(d2V)
  Subsystem4/1(M) -> [M]
  [dlty] -> Subsystem3/1(dlty)
  [mach] -> Subsystem3/2(Mach)
  [qsd] -> Subsystem3/4(qSd)
  [r] -> Subsystem3/5(r)
  [d2v] -> Subsystem3/6(d2V)
  Subsystem3/1(N) -> [N]
  [Fx] -> Mux/1
  [Fy] -> Mux/2
  [Fz] -> Mux/3
  [L] -> Mux1/1
  [M] -> Mux1/2
  [N] -> Mux1/3
  dlty/1 -> [dlty]
  dltz/1 -> [dltz]
  Demux/1 -> Terminator4/1
  Demux/2 -> [q]
  Demux/3 -> [r]
  [r] -> Subsystem1/6(r)
  Constant1/1 -> [L]
  [betap] -> Subsystem1/7(betap)
  [betap] -> Subsystem3/7(betap)

== system AED2D/Dinâmica 6DOF/Gravidade ==
  DCM : Inport
  Constant1 : Constant  Value=D.m
  Constant2 : Constant  Value=0
  Constant3 : Constant  Value=0
  Constant4 : Constant  Value=g
  Mux : Mux  Inputs=3
  Product : Product
  "transform to Inertial axes " : shared6dof/6DOF (Euler Angles)/transform to Inertial axes   SystemSampleTime=-1
      settings: SourceProductName=Aerospace Blockset  SourceProductBaseCode=AE
  Fg_b : Outport
  g_b : Outport  Port=2
  wires:
  Constant3/1 -> Mux/2
  Constant2/1 -> Mux/1
  Constant4/1 -> Mux/3
  Constant1/1 -> Product/2
  Mux/1 -> g_b/1, Product/1
  DCM/1 -> "transform to Inertial axes "/2
  Product/1 -> "transform to Inertial axes "/1
  "transform to Inertial axes "/1 -> Fg_b/1

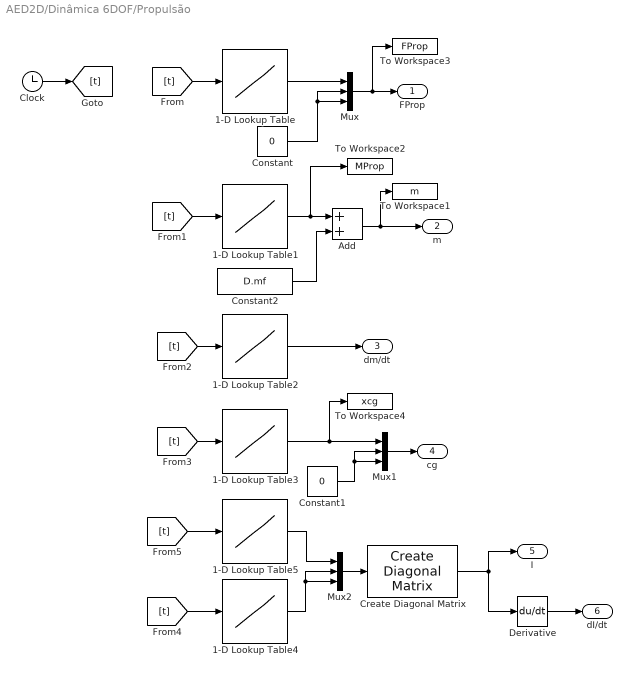
== system AED2D/Dinâmica 6DOF/Propulsão ==
  1-D Lookup Table : Lookup_n-D  NumberOfTableDimensions=1  BreakpointsForDimension1="[0  D.T_propB   D.T_propB+0.001  (D.T_propS+D.T_propB)   (D.T_propS+D.T_propB+0.001)]"  Table="[D.F_propB   D. F_propB   D. F_propS  D.F_propS  0]"  ExtrapMethod=Clip  InternalRulePriority=Speed  RndMeth=Simplest  InputSameDT=on
  1-D Lookup Table1 : Lookup_n-D  NumberOfTableDimensions=1  BreakpointsForDimension1="[0  D.T_propB+D.T_propS  D.T_propB+D.T_propS+0.001]"  Table="[D.m_prop0    0   0]"  ExtrapMethod=Clip  InternalRulePriority=Speed  RndMeth=Simplest  InputSameDT=on
  1-D Lookup Table2 : Lookup_n-D  NumberOfTableDimensions=1  BreakpointsForDimension1="[0  D.T_propB  D.T_propB+0.001  (D.T_propB+D.T_propS)  (D.T_propB+D.T_propS+0.001)]"  Table="[D.dmdtB  D.dmdtB  D.dmdtS  D.dmdtS  0]"  ExtrapMethod=Clip  InternalRulePriority=Speed  RndMeth=Simplest  InputSameDT=on
  1-D Lookup Table3 : Lookup_n-D  NumberOfTableDimensions=1  BreakpointsForDimension1="[0  D.T_propB/2  D.T_propB  (D.T_propB+D.T_propS/2)  (D.T_propB+D.T_propS)]"  Table="[D.xcg0  D.xcgBm  D.xcgBf  D.xcgSm  D.xcgf]"  ExtrapMethod=Clip  InternalRulePriority=Speed  RndMeth=Simplest  InputSameDT=on
  1-D Lookup Table4 : Lookup_n-D  NumberOfTableDimensions=1  BreakpointsForDimension1="[0  D.T_propB/2  D.T_propB  (D.T_propB+D.T_propS/2)  (D.T_propB+D.T_propS)]"  Table="[D.Iy0  D.IyBm  D.IyBf  D.IySm  D.Iyf]"  ExtrapMethod=Clip  InternalRulePriority=Speed  RndMeth=Simplest  InputSameDT=on
  1-D Lookup Table5 : Lookup_n-D  NumberOfTableDimensions=1  BreakpointsForDimension1="[0  D.T_propB/2  D.T_propB  (D.T_propB+D.T_propS/2)  (D.T_propB+D.T_propS)]"  Table="[D.Ix0  D.IxBm  D.IxBf  D.IxSm  D.Ixf]"  ExtrapMethod=Clip  InternalRulePriority=Speed  RndMeth=Simplest  InputSameDT=on
  Add : Sum
  Clock : Clock
  Constant : Constant  Value=0
  Constant1 : Constant  Value=0
  Constant2 : Constant  Value=D.mf
  Create Diagonal Matrix : dspmtrx3/Create Diagonal Matrix
      settings: SourceProductName=DSP System Toolbox  SourceProductBaseCode=DS
  Derivative : Derivative
  Mux : Mux  Inputs=3
  Mux1 : Mux  Inputs=3
  Mux2 : Mux  Inputs=3
  To Workspace1 : ToWorkspace  VariableName=m  SaveFormat=Timeseries  SampleTime=-1
  To Workspace2 : ToWorkspace  VariableName=MProp  SaveFormat=Timeseries  SampleTime=-1
  To Workspace3 : ToWorkspace  VariableName=FProp  SaveFormat=Timeseries  SampleTime=-1
  To Workspace4 : ToWorkspace  VariableName=xcg  SaveFormat=Timeseries  SampleTime=-1
  FProp : Outport
  m : Outport  Port=2
  dm/dt : Outport  Port=3
  cg : Outport  Port=4
  I : Outport  Port=5
  dI/dt : Outport  Port=6
  wires:
  Mux/1 -> FProp/1, To Workspace3/1
  1-D Lookup Table/1 -> Mux/1
  Constant/1 -> Mux/3, Mux/2
  1-D Lookup Table1/1 -> To Workspace2/1, Add/1
  1-D Lookup Table2/1 -> dm/dt/1
  Add/1 -> m/1, To Workspace1/1
  Constant2/1 -> Add/2
  Derivative/1 -> dI/dt/1
  Mux1/1 -> cg/1
  1-D Lookup Table3/1 -> To Workspace4/1, Mux1/1
  Constant1/1 -> Mux1/2, Mux1/3
  Create Diagonal Matrix/1 -> I/1, Derivative/1
  1-D Lookup Table5/1 -> Mux2/1
  1-D Lookup Table4/1 -> Mux2/3, Mux2/2
  Mux2/1 -> Create Diagonal Matrix/1
  Clock/1 -> [t]
  [t] -> 1-D Lookup Table/1
  [t] -> 1-D Lookup Table1/1
  [t] -> 1-D Lookup Table2/1
  [t] -> 1-D Lookup Table3/1
  [t] -> 1-D Lookup Table4/1
  [t] -> 1-D Lookup Table5/1

== system AED2D/Guiamento/Controle de Atitude ==
  Xe : Inport
  AP : Inport  Port=2
  " " : Switch  Criteria=u2 > Threshold
  " 1" : Switch  Criteria=u2 > Threshold  Threshold=TTrav
  " 2" : Switch  Criteria=u2 > Threshold  Threshold=TTrav
  Clock : Clock
  Constant2 : Constant  Value=0
  Constant3 : Constant  Value=AltCruz
  Constant4 : Constant  Value=atan(Ya0/Xa0)
  Demux1 : Demux  Outputs=3
  Gain : Gain  Gain=GanhoAtit
  Saturation1 : Saturate  UpperLimit=RampaMax  LowerLimit=-RampaMax
  Sum : Sum  Inputs=|+-
  Terminator1 : Terminator
  Terminator4 : Terminator
  To Workspace : ToWorkspace  VariableName=PsiRef  SaveFormat=Timeseries  SampleTime=-1
  To Workspace1 : ToWorkspace  VariableName=ThetaRef  SaveFormat=Timeseries  SampleTime=-1
  To Workspace2 : ToWorkspace  VariableName=altdiff  SaveFormat=Timeseries  SampleTime=-1
  psiREF : Outport
  ThetaRef : Outport  Port=2
  wires:
  Xe/1 -> Demux1/1
  AP/1 -> " "/2
  Constant3/1 -> Sum/2
  Demux1/3 -> Sum/1
  Demux1/2 -> Terminator4/1
  Demux1/1 -> Terminator1/1
  Clock/1 -> " 1"/2, " 2"/2
  Constant2/1 -> " "/1, " 2"/3, " 1"/3
  " "/1 -> " 1"/1
  " 1"/1 -> ThetaRef/1, To Workspace1/1
  Constant4/1 -> " 2"/1
  " 2"/1 -> To Workspace/1, psiREF/1
  Saturation1/1 -> " "/3
  Sum/1 -> To Workspace2/1, Gain/1
  Gain/1 -> Saturation1/1

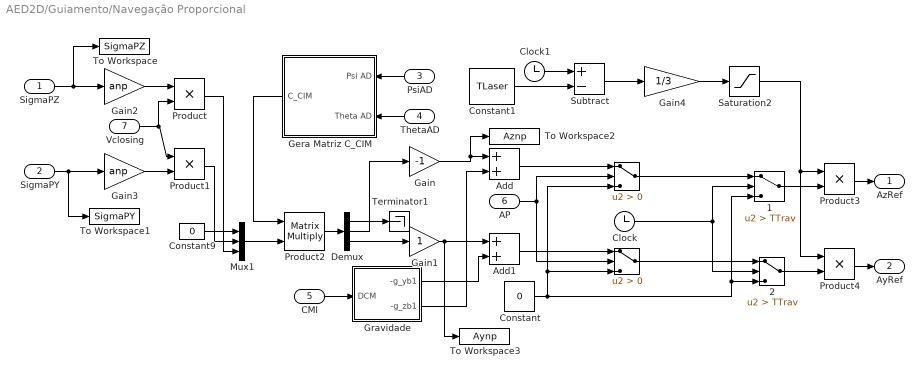
== system AED2D/Guiamento/Navegação Proporcional  ==
  SigmaPZ : Inport
  SigmaPY : Inport  Port=2
  PsiAD : Inport  Port=3
  ThetaAD : Inport  Port=4
  CMI : Inport  Port=5
  AP : Inport  Port=6
  Vclosing : Inport  Port=7
  " " : Switch  Criteria=u2 > Threshold
  "  " : Switch  Criteria=u2 > Threshold
  " 1" : Switch  Criteria=u2 > Threshold  Threshold=TTrav
  " 2" : Switch  Criteria=u2 > Threshold  Threshold=TTrav
  Add : Sum
  Add1 : Sum
  Clock : Clock
  Clock1 : Clock
  Constant : Constant  Value=0
  Constant1 : Constant  Value=TLaser
  Constant9 : Constant  Value=0
  Demux : Demux  Outputs=3
  Gain : Gain  Gain=-1
  Gain1 : Gain
  Gain2 : Gain  Gain=anp
  Gain3 : Gain  Gain=anp
  Gain4 : Gain  Gain=1/3
  Gera Matriz C_CIM : Subsystem
  Gravidade : Subsystem
  Mux1 : Mux  Inputs=3
  Product{,1,3..4} (4 alike) : Product
  Product2 : Product  Multiplication=Matrix(*)
  Saturation2 : Saturate  UpperLimit=1  LowerLimit=0
  Subtract : Sum  Inputs=+-
  Terminator1 : Terminator
  To Workspace : ToWorkspace  VariableName=SigmaPZ  SaveFormat=Timeseries  SampleTime=-1
  To Workspace1 : ToWorkspace  VariableName=SigmaPY  SaveFormat=Timeseries  SampleTime=-1
  To Workspace2 : ToWorkspace  VariableName=Aznp  SaveFormat=Timeseries  SampleTime=-1
  To Workspace3 : ToWorkspace  VariableName=Aynp  SaveFormat=Timeseries  SampleTime=-1
  AzRef : Outport
  AyRef : Outport  Port=2
  wires:
  Demux/1 -> Terminator1/1
  Mux1/1 -> Product2/2
  CMI/1 -> Gravidade/1(DCM)
  Product2/1 -> Demux/1
  SigmaPY/1 -> Gain3/1, To Workspace1/1
  Gain1/1 -> Add1/1, To Workspace3/1
  Gain/1 -> To Workspace2/1, Add/1
  Constant9/1 -> Mux1/1
  AP/1 -> "  "/2, " "/2
  Add/1 -> " "/1
  Add1/1 -> "  "/1
  Gera Matriz C_CIM/1(C_CIM) -> Product2/1
  SigmaPZ/1 -> Gain2/1, To Workspace/1
  Gravidade/1(-g_yb1) -> Add1/2
  Gravidade/2(-g_zb1) -> Add/2
  " "/1 -> " 1"/1
  Clock/1 -> " 2"/2, " 1"/2
  Constant/1 -> " 1"/3, " 2"/3, " "/3, "  "/3
  "  "/1 -> " 2"/1
  Vclosing/1 -> Product1/1, Product/2
  Product/1 -> Mux1/3
  Gain3/1 -> Product1/2
  Product1/1 -> Mux1/2
  Constant1/1 -> Subtract/2
  Subtract/1 -> Gain4/1
  Gain4/1 -> Saturation2/1
  Clock1/1 -> Subtract/1
  Saturation2/1 -> Product3/1, Product4/1
  " 1"/1 -> Product3/2
  " 2"/1 -> Product4/2
  Gain2/1 -> Product/1
  Product3/1 -> AzRef/1
  Product4/1 -> AyRef/1
  PsiAD/1 -> Gera Matriz C_CIM/1(Psi AD)
  ThetaAD/1 -> Gera Matriz C_CIM/2(Theta AD)
  Demux/3 -> Gain1/1
  Demux/2 -> Gain/1

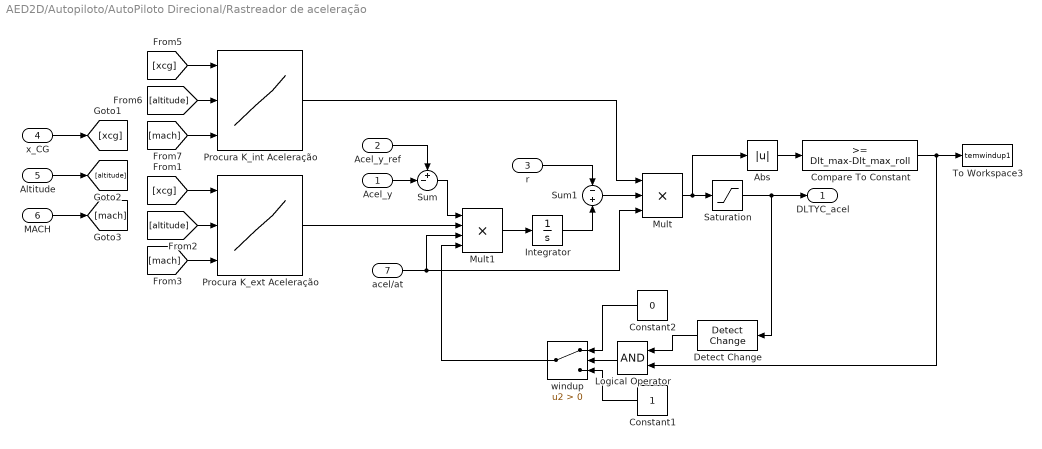
== system AED2D/Autopiloto/AutoPiloto Direcional/Rastreador de aceleração ==
  Acel_y : Inport
  Acel_y_ref : Inport  Port=2
  r : Inport  Port=3
  x_CG : Inport  Port=4
  Altitude : Inport  Port=5
  MACH : Inport  Port=6
  acel/at : Inport  Port=7
  Abs : Abs
  Compare To Constant : simulink/Logic and Bit Operations/Compare To Constant  relop=>=  const=Dlt_max-Dlt_max_roll  OutDataTypeStr=boolean
  Constant1 : Constant
  Constant2 : Constant  Value=0
  Detect Change : simulink/Logic and Bit Operations/Detect Change  vinit=0  OutDataTypeStr=boolean
  Integrator : Integrator  UpperSaturationLimit=sat_integAP  LowerSaturationLimit=-sat_integAP
  Logical Operator : Logic  AllPortsSameDT=off  OutDataTypeStr=boolean
  Mult : Product  Inputs=***
  Mult1 : Product  Inputs=****
  Procura K_ext Aceleração : Lookup_n-D  NumberOfTableDimensions=3  BreakpointsForDimension1=vet_x_CG  BreakpointsForDimension2=vet_altitude  BreakpointsForDimension3=vet_Mach  Table=T_acel_k_ext  ExtrapMethod=Clip  InternalRulePriority=Speed  RndMeth=Simplest  InputSameDT=on
  Procura K_int Aceleração : Lookup_n-D  NumberOfTableDimensions=3  BreakpointsForDimension1=vet_x_CG  BreakpointsForDimension2=vet_altitude  BreakpointsForDimension3=vet_Mach  Table=T_acel_k_int  ExtrapMethod=Clip  InternalRulePriority=Speed  RndMeth=Simplest  InputSameDT=on
  Saturation : Saturate  UpperLimit=Dlt_max-Dlt_max_roll  LowerLimit=-Dlt_max+Dlt_max_roll
  Sum : Sum  Inputs=+-|
  Sum1 : Sum  Inputs=-+
  To Workspace3 : ToWorkspace  VariableName=temwindup1  SaveFormat=Timeseries  SampleTime=-1
  windup : Switch  Criteria=u2 > Threshold
  DLTYC_acel : Outport
  wires:
  Constant1/1 -> windup/3
  Logical Operator/1 -> windup/2
  Altitude/1 -> [altitude]
  Saturation/1 -> Detect Change/1, DLTYC_acel/1
  Acel_y/1 -> Sum/2
  [altitude] -> Procura K_int Aceleração/2
  Mult1/1 -> Integrator/1
  Abs/1 -> Compare To Constant/1
  acel/at/1 -> Mult/3, Mult1/3
  Detect Change/1 -> Logical Operator/1
  Constant2/1 -> windup/1
  windup/1 -> Mult1/4
  Procura K_ext Aceleração/1 -> Mult1/2
  [mach] -> Procura K_int Aceleração/3
  [xcg] -> Procura K_ext Aceleração/1
  [xcg] -> Procura K_int Aceleração/1
  Mult/1 -> Abs/1, Saturation/1
  x_CG/1 -> [xcg]
  MACH/1 -> [mach]
  Sum/1 -> Mult1/1
  [altitude] -> Procura K_ext Aceleração/2
  [mach] -> Procura K_ext Aceleração/3
  Compare To Constant/1 -> Logical Operator/2, To Workspace3/1
  Acel_y_ref/1 -> Sum/1
  Sum1/1 -> Mult/2
  Procura K_int Aceleração/1 -> Mult/1
  Integrator/1 -> Sum1/2
  r/1 -> Sum1/1

== system AED2D/Autopiloto/AutoPiloto Direcional/Rastreador de atitude ==
  r : Inport
  x_CG : Inport  Port=2
  Altitude : Inport  Port=3
  MACH : Inport  Port=4
  Psi : Inport  Port=5
  Psi_ref : Inport  Port=6
  Mult : Product  Inputs=**
  Mult1 : Product  Inputs=**
  Procura K_ext Atitude : Lookup_n-D  NumberOfTableDimensions=3  BreakpointsForDimension1=vet_x_CG  BreakpointsForDimension2=vet_altitude  BreakpointsForDimension3=vet_Mach  Table=T_at_k_ext  ExtrapMethod=Clip  InternalRulePriority=Speed  RndMeth=Simplest  InputSameDT=on
  Procura K_int Atitude : Lookup_n-D  NumberOfTableDimensions=3  BreakpointsForDimension1=vet_x_CG  BreakpointsForDimension2=vet_altitude  BreakpointsForDimension3=vet_Mach  Table=T_at_k_int  ExtrapMethod=Clip  InternalRulePriority=Speed  RndMeth=Simplest  InputSameDT=on
  Saturation : Saturate  UpperLimit=Dlt_max-Dlt_max_roll  LowerLimit=-Dlt_max+Dlt_max_roll
  Sum : Sum  Inputs=|+-
  Sum1 : Sum  Inputs=-+
  DLTYC_atitude : Outport
  wires:
  Mult1/1 -> Sum1/2
  Procura K_int Atitude/1 -> Mult/1
  r/1 -> Sum1/1
  x_CG/1 -> [xcg]
  Altitude/1 -> [altitude]
  MACH/1 -> [mach]
  [xcg] -> Procura K_int Atitude/1
  [altitude] -> Procura K_int Atitude/2
  [mach] -> Procura K_int Atitude/3
  [xcg] -> Procura K_ext Atitude/1
  [altitude] -> Procura K_ext Atitude/2
  [mach] -> Procura K_ext Atitude/3
  Saturation/1 -> DLTYC_atitude/1
  Sum1/1 -> Mult/2
  Mult/1 -> Saturation/1
  Psi/1 -> Sum/2
  Psi_ref/1 -> Sum/1
  Procura K_ext Atitude/1 -> Mult1/1
  Sum/1 -> Mult1/2

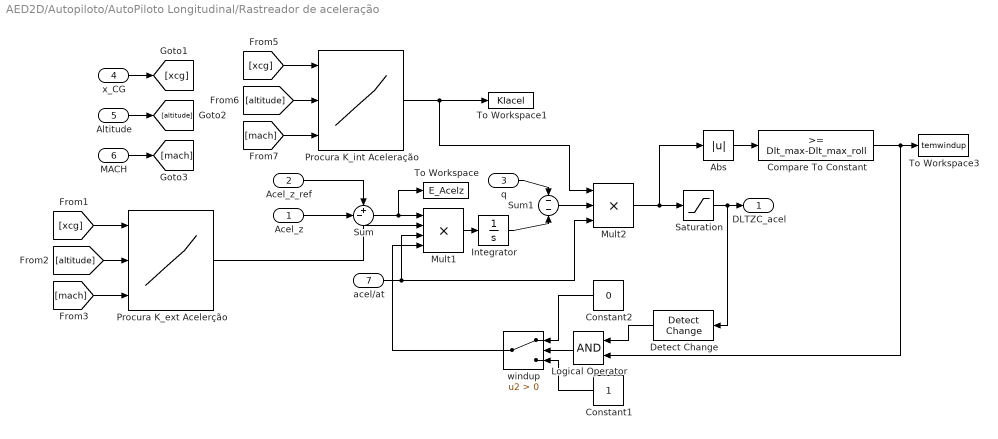
== system AED2D/Autopiloto/AutoPiloto Longitudinal/Rastreador de aceleração ==
  Acel_z : Inport
  Acel_z_ref : Inport  Port=2
  q : Inport  Port=3
  x_CG : Inport  Port=4
  Altitude : Inport  Port=5
  MACH : Inport  Port=6
  acel/at : Inport  Port=7
  Abs : Abs
  Compare To Constant : simulink/Logic and Bit Operations/Compare To Constant  relop=>=  const=Dlt_max-Dlt_max_roll  OutDataTypeStr=boolean
  Constant1 : Constant
  Constant2 : Constant  Value=0
  Detect Change : simulink/Logic and Bit Operations/Detect Change  vinit=0  OutDataTypeStr=boolean
  Integrator : Integrator  UpperSaturationLimit=sat_integAP  LowerSaturationLimit=-sat_integAP
  Logical Operator : Logic  AllPortsSameDT=off  OutDataTypeStr=boolean
  Mult1 : Product  Inputs=****
  Mult2 : Product  Inputs=***
  Procura K_ext Acelerção : Lookup_n-D  NumberOfTableDimensions=3  BreakpointsForDimension1=vet_x_CG  BreakpointsForDimension2=vet_altitude  BreakpointsForDimension3=vet_Mach  Table=T_acel_k_ext  ExtrapMethod=Clip  InternalRulePriority=Speed  RndMeth=Simplest  InputSameDT=on
  Procura K_int Aceleração : Lookup_n-D  NumberOfTableDimensions=3  BreakpointsForDimension1=vet_x_CG  BreakpointsForDimension2=vet_altitude  BreakpointsForDimension3=vet_Mach  Table=T_acel_k_int  ExtrapMethod=Clip  InternalRulePriority=Speed  RndMeth=Simplest  InputSameDT=on
  Saturation : Saturate  UpperLimit=Dlt_max-Dlt_max_roll  LowerLimit=-Dlt_max+Dlt_max_roll
  Sum : Sum  Inputs=+-|
  Sum1 : Sum  Inputs=--
  To Workspace : ToWorkspace  VariableName=E_Acelz  SaveFormat=Timeseries  SampleTime=-1
  To Workspace1 : ToWorkspace  VariableName=KIacel  SaveFormat=Timeseries  SampleTime=-1
  To Workspace3 : ToWorkspace  VariableName=temwindup  SaveFormat=Timeseries  SampleTime=-1
  windup : Switch  Criteria=u2 > Threshold
  DLTZC_acel : Outport
  wires:
  Mult2/1 -> Abs/1, Saturation/1
  Sum1/1 -> Mult2/2
  Compare To Constant/1 -> Logical Operator/2, To Workspace3/1
  Logical Operator/1 -> windup/2
  [altitude] -> Procura K_ext Acelerção/2
  acel/at/1 -> Mult2/3, Mult1/3
  Procura K_ext Acelerção/1 -> Mult1/2
  [altitude] -> Procura K_int Aceleração/2
  [xcg] -> Procura K_int Aceleração/1
  x_CG/1 -> [xcg]
  [mach] -> Procura K_int Aceleração/3
  Altitude/1 -> [altitude]
  Sum/1 -> To Workspace/1, Mult1/1
  Acel_z/1 -> Sum/2
  q/1 -> Sum1/1
  Mult1/1 -> Integrator/1
  Abs/1 -> Compare To Constant/1
  Integrator/1 -> Sum1/2
  MACH/1 -> [mach]
  [mach] -> Procura K_ext Acelerção/3
  Procura K_int Aceleração/1 -> Mult2/1, To Workspace1/1
  Detect Change/1 -> Logical Operator/1
  windup/1 -> Mult1/4
  Acel_z_ref/1 -> Sum/1
  Saturation/1 -> Detect Change/1, DLTZC_acel/1
  [xcg] -> Procura K_ext Acelerção/1
  Constant2/1 -> windup/1
  Constant1/1 -> windup/3

== system AED2D/Autopiloto/AutoPiloto Longitudinal/Rastreador de atitude ==
  Theta : Inport
  Theta_ref : Inport  Port=2
  q : Inport  Port=3
  x_CG : Inport  Port=4
  Altitude : Inport  Port=5
  MACH : Inport  Port=6
  Mult : Product  Inputs=**
  Mult1 : Product  Inputs=**
  Procura K_ext Atitude : Lookup_n-D  NumberOfTableDimensions=3  BreakpointsForDimension1=vet_x_CG  BreakpointsForDimension2=vet_altitude  BreakpointsForDimension3=vet_Mach  Table=T_at_k_ext  ExtrapMethod=Clip  InternalRulePriority=Speed  RndMeth=Simplest  InputSameDT=on
  Procura K_int Atitude : Lookup_n-D  NumberOfTableDimensions=3  BreakpointsForDimension1=vet_x_CG  BreakpointsForDimension2=vet_altitude  BreakpointsForDimension3=vet_Mach  Table=T_at_k_int  ExtrapMethod=Clip  InternalRulePriority=Speed  RndMeth=Simplest  InputSameDT=on
  Saturation : Saturate  UpperLimit=Dlt_max-Dlt_max_roll  LowerLimit=-Dlt_max+Dlt_max_roll
  Sum : Sum  Inputs=|+-
  Sum1 : Sum  Inputs=|+-
  DLTZC_atitude : Outport
  wires:
  Procura K_int Atitude/1 -> Mult/1
  x_CG/1 -> [xcg]
  Altitude/1 -> [altitude]
  MACH/1 -> [mach]
  [xcg] -> Procura K_int Atitude/1
  [altitude] -> Procura K_int Atitude/2
  [mach] -> Procura K_int Atitude/3
  [mach] -> Procura K_ext Atitude/3
  [altitude] -> Procura K_ext Atitude/2
  [xcg] -> Procura K_ext Atitude/1
  Saturation/1 -> DLTZC_atitude/1
  Sum1/1 -> Mult/2
  Mult/1 -> Saturation/1
  q/1 -> Sum1/2
  Mult1/1 -> Sum1/1
  Theta/1 -> Sum/2
  Theta_ref/1 -> Sum/1
  Procura K_ext Atitude/1 -> Mult1/1
  Sum/1 -> Mult1/2
